simulink model "ConstructionCradleControl"  (R2023a)
settings: Solver=ode23tb  StartTime=0.0  StopTime=100  FixedStep=1e-3  RelTol=1e-3
model workspace (MAT data in the model file):
  ReqValues_3.Name = 'StepRespEnvelope'
  ReqValues_3.Type = '<='
  ReqValues_3.Value = [-0.861893287814; -0.774378435339; -0.00986894621533; -1; 0.873403601496; 0.846548097571; 0.769820423932; 328.086118526]
  ReqValues_3.DisplayValue = [-0.861893287814; -0.774378435339; -0.00986894621533; -1; 0.873403601496; 0.846548097571; 0.769820423932; 328.086118526]
  ReqValues_3_1.Name = 'StepRespEnvelope'
  ReqValues_3_1.Type = '<='
  ReqValues_3_1.Value = [-0.861893287814; -0.774378435339; -0.00986894621533; -1; 0.873403601496; 0.846548097571; 0.769820423932; 328.086118526]
  ReqValues_3_1.DisplayValue = [-0.861893287814; -0.774378435339; -0.00986894621533; -1; 0.873403601496; 0.846548097571; 0.769820423932; 328.086118526]
settings Model: Creator=Ilya_Andriyanov  LastModifiedBy=ycheb

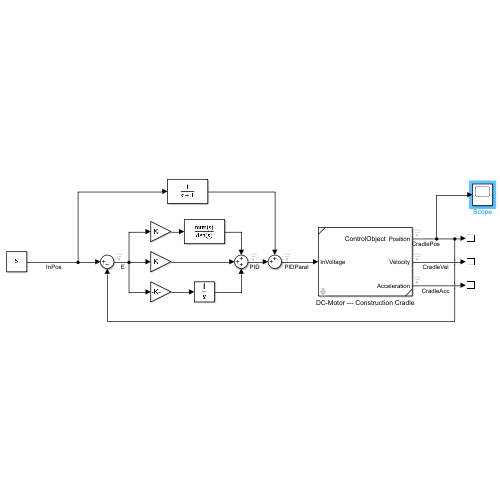
[thumbnail: Simulink's stored preview of the top-level diagram]
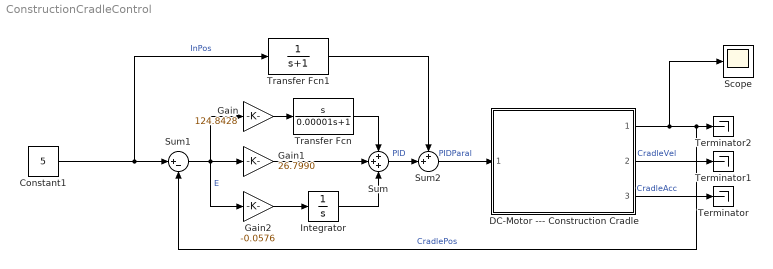
== system ConstructionCradleControl ==
  Constant1 : Constant  Value=5
  DC-Motor --- Construction Cradle : Subsystem  ReferencedSubsystem=ControlObject  motor_nominal_voltage=24  L=300e-6  R=8.5  km=17e-1  kw=17e-2  J_motor=500e-9  vis_friction_coef_motor=0.001  i_gear=200  J_gear=2.4e-9  vis_friction_coef_gear=0.001  r_cyl=0.3  vis_friction_coef_cradle=0.001  cradle_mass=5
  Gain : Gain  Gain=124.8428
  Gain1 : Gain  Gain=26.7990
  Gain2 : Gain  Gain=-0.0576
  Integrator : Integrator
  Scope : Scope
  Sum : Sum  Inputs=+++
  Sum1 : Sum  Inputs=|+-
  Sum2 : Sum  Inputs=++|
  Terminator : Terminator
  Terminator1 : Terminator
  Terminator2 : Terminator
  Transfer Fcn : TransferFcn  Numerator=[1 0]  Denominator=[0.00001 1]
  Transfer Fcn1 : TransferFcn  Denominator=[1 1]
  wires:
  DC-Motor --- Construction Cradle/1 -> Scope/1, Sum1/2, Terminator2/1  "CradlePos"
  DC-Motor --- Construction Cradle/2 -> Terminator1/1  "CradleVel"
  DC-Motor --- Construction Cradle/3 -> Terminator/1  "CradleAcc"
  Gain/1 -> Transfer Fcn/1
  Gain2/1 -> Integrator/1
  Gain1/1 -> Sum/2
  Transfer Fcn/1 -> Sum/1
  Integrator/1 -> Sum/3
  Sum1/1 -> Gain2/1, Gain/1, Gain1/1  "E"
  Sum/1 -> Sum2/2  "PID"
  Transfer Fcn1/1 -> Sum2/1
  Constant1/1 -> Transfer Fcn1/1, Sum1/1  "InPos"
  Sum2/1 -> DC-Motor --- Construction Cradle/1  "PIDParal"
